simulink model "TanqueNL"  (R2020a)
settings: Solver=VariableStepAuto  StartTime=0.0  StopTime=20  RelTol=1e-3
undefined symbols (not defined in the file or in its folder): h0
settings Model: Creator=a1  LastModifiedBy=a1

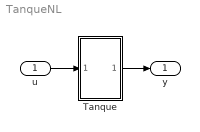
== system TanqueNL ==
  u : Inport
  Tanque : Subsystem
  y : Outport
  wires:
  Tanque/1(h(t)) -> y/1
  u/1 -> Tanque/1(e(t))

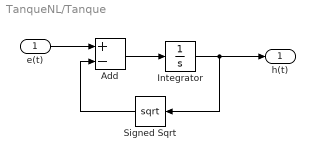
== system TanqueNL/Tanque ==
  e(t) : Inport
  Add : Sum  Inputs=+-
  Integrator : Integrator  InitialCondition=h0
  Signed Sqrt : Sqrt  OutputSignalType=real  SaturateOnIntegerOverflow=on
  h(t) : Outport
  wires:
  e(t)/1 -> Add/1
  Signed Sqrt/1 -> Add/2
  Add/1 -> Integrator/1
  Integrator/1 -> h(t)/1, Signed Sqrt/1
